simulink model "top_level_algo"  (R2022b)
settings: Solver=FixedStepAuto  StartTime=0.0  StopTime=inf  FixedStep=1e-3  RelTol=1e-3
values from neighbouring files (symbols this model uses):
  clk_period = 8    [Cals.m]
  gear_ratio = 10    [Cals.m]
  update_rate = 0.5    [Cals.m]
  Vdd = 3    [Cals.m]
undefined symbols (not defined in the file or in its folder): sigbuilder_block
libraries: simulink x24, stm32f4xxblockslib x12, embmathops x9, arduinolib x8, dspstat3 x4, dspswit3 x2
(part 3 of 3)

== system top_level_algo/7seg Driver2/HR Encoding/7seg encoder2/If Action Subsystem10 ==
  Action Port : ActionPort  ActionPortLabel=case [ 9 ]:
  Constant : Constant  Value=0x6F
  Out1 : Outport
  wires:
  Constant/1 -> Out1/1

== system top_level_algo/7seg Driver2/HR Encoding/7seg encoder2/If Action Subsystem2 ==
  Action Port : ActionPort  ActionPortLabel=case [ 2 ]:
  Constant : Constant  Value=0x5B
  Out1 : Outport
  wires:
  Constant/1 -> Out1/1

== system top_level_algo/7seg Driver2/HR Encoding/7seg encoder2/If Action Subsystem3 ==
  Action Port : ActionPort  ActionPortLabel=case [ 3 ]:
  Constant : Constant  Value=0x4F
  Out1 : Outport
  wires:
  Constant/1 -> Out1/1

== system top_level_algo/7seg Driver2/HR Encoding/7seg encoder2/If Action Subsystem4 ==
  Action Port : ActionPort  ActionPortLabel=case [ 4 ]:
  Constant : Constant  Value=0x66
  Out1 : Outport
  wires:
  Constant/1 -> Out1/1

== system top_level_algo/7seg Driver2/HR Encoding/7seg encoder2/If Action Subsystem5 ==
  Action Port : ActionPort  ActionPortLabel=case [ 5 ]:
  Constant : Constant  Value=0x6D
  Out1 : Outport
  wires:
  Constant/1 -> Out1/1

== system top_level_algo/7seg Driver2/HR Encoding/7seg encoder2/If Action Subsystem6 ==
  Action Port : ActionPort  ActionPortLabel=case [ 6 ]:
  Constant : Constant  Value=0x7D
  Out1 : Outport
  wires:
  Constant/1 -> Out1/1

== system top_level_algo/7seg Driver2/HR Encoding/7seg encoder2/If Action Subsystem7 ==
  Action Port : ActionPort  ActionPortLabel=case [ 7 ]:
  Constant : Constant  Value=0x07
  Out1 : Outport
  wires:
  Constant/1 -> Out1/1

== system top_level_algo/7seg Driver2/HR Encoding/7seg encoder2/If Action Subsystem8 ==
  Action Port : ActionPort  ActionPortLabel=case [ 8 ]:
  Constant : Constant  Value=0x7F
  Out1 : Outport
  wires:
  Constant/1 -> Out1/1

== system top_level_algo/7seg Driver2/HR Encoding/old encoder3/If Action Subsystem ==
  Action Port : ActionPort
  Constant : Constant  Value=0x3F
  Out1 : Outport
  wires:
  Constant/1 -> Out1/1

== system top_level_algo/7seg Driver2/HR Encoding/old encoder3/If Action Subsystem1 ==
  Action Port : ActionPort
  Constant : Constant  Value=0x06
  Out1 : Outport
  wires:
  Constant/1 -> Out1/1

== system top_level_algo/7seg Driver2/HR Encoding/old encoder3/If Action Subsystem10 ==
  Action Port : ActionPort
  Constant : Constant  Value=0x6F
  Out1 : Outport
  wires:
  Constant/1 -> Out1/1

== system top_level_algo/7seg Driver2/HR Encoding/old encoder3/If Action Subsystem2 ==
  Action Port : ActionPort
  Constant : Constant  Value=0x5B
  Out1 : Outport
  wires:
  Constant/1 -> Out1/1

== system top_level_algo/7seg Driver2/HR Encoding/old encoder3/If Action Subsystem3 ==
  Action Port : ActionPort
  Constant : Constant  Value=0x4F
  Out1 : Outport
  wires:
  Constant/1 -> Out1/1

== system top_level_algo/7seg Driver2/HR Encoding/old encoder3/If Action Subsystem4 ==
  Action Port : ActionPort
  Constant : Constant  Value=0x66
  Out1 : Outport
  wires:
  Constant/1 -> Out1/1

== system top_level_algo/7seg Driver2/HR Encoding/old encoder3/If Action Subsystem5 ==
  Action Port : ActionPort
  Constant : Constant  Value=0x6D
  Out1 : Outport
  wires:
  Constant/1 -> Out1/1

== system top_level_algo/7seg Driver2/HR Encoding/old encoder3/If Action Subsystem6 ==
  Action Port : ActionPort
  Constant : Constant  Value=0x7D
  Out1 : Outport
  wires:
  Constant/1 -> Out1/1

== system top_level_algo/7seg Driver2/HR Encoding/old encoder3/If Action Subsystem7 ==
  Action Port : ActionPort
  Constant : Constant  Value=0x07
  Out1 : Outport
  wires:
  Constant/1 -> Out1/1

== system top_level_algo/7seg Driver2/HR Encoding/old encoder3/If Action Subsystem8 ==
  Action Port : ActionPort
  Constant : Constant  Value=0x7F
  Out1 : Outport
  wires:
  Constant/1 -> Out1/1

== system top_level_algo/Speed up 7seg Driver/HR Encoding/7seg encoder/If Action Subsystem ==
  Action Port : ActionPort  ActionPortLabel=case [ 0 ]:
  Constant : Constant  Value=0x3F
  Out1 : Outport
  wires:
  Constant/1 -> Out1/1

== system top_level_algo/Speed up 7seg Driver/HR Encoding/7seg encoder/If Action Subsystem1 ==
  Action Port : ActionPort  ActionPortLabel=case [ 1 ]:
  Constant : Constant  Value=0x06
  Out1 : Outport
  wires:
  Constant/1 -> Out1/1

== system top_level_algo/Speed up 7seg Driver/HR Encoding/7seg encoder/If Action Subsystem10 ==
  Action Port : ActionPort  ActionPortLabel=case [ 9 ]:
  Constant : Constant  Value=0x6F
  Out1 : Outport
  wires:
  Constant/1 -> Out1/1

== system top_level_algo/Speed up 7seg Driver/HR Encoding/7seg encoder/If Action Subsystem2 ==
  Action Port : ActionPort  ActionPortLabel=case [ 2 ]:
  Constant : Constant  Value=0x5B
  Out1 : Outport
  wires:
  Constant/1 -> Out1/1

== system top_level_algo/Speed up 7seg Driver/HR Encoding/7seg encoder/If Action Subsystem3 ==
  Action Port : ActionPort  ActionPortLabel=case [ 3 ]:
  Constant : Constant  Value=0x4F
  Out1 : Outport
  wires:
  Constant/1 -> Out1/1

== system top_level_algo/Speed up 7seg Driver/HR Encoding/7seg encoder/If Action Subsystem4 ==
  Action Port : ActionPort  ActionPortLabel=case [ 4 ]:
  Constant : Constant  Value=0x66
  Out1 : Outport
  wires:
  Constant/1 -> Out1/1

== system top_level_algo/Speed up 7seg Driver/HR Encoding/7seg encoder/If Action Subsystem5 ==
  Action Port : ActionPort  ActionPortLabel=case [ 5 ]:
  Constant : Constant  Value=0x6D
  Out1 : Outport
  wires:
  Constant/1 -> Out1/1

== system top_level_algo/Speed up 7seg Driver/HR Encoding/7seg encoder/If Action Subsystem6 ==
  Action Port : ActionPort  ActionPortLabel=case [ 6 ]:
  Constant : Constant  Value=0x7D
  Out1 : Outport
  wires:
  Constant/1 -> Out1/1

== system top_level_algo/Speed up 7seg Driver/HR Encoding/7seg encoder/If Action Subsystem7 ==
  Action Port : ActionPort  ActionPortLabel=case [ 7 ]:
  Constant : Constant  Value=0x07
  Out1 : Outport
  wires:
  Constant/1 -> Out1/1

== system top_level_algo/Speed up 7seg Driver/HR Encoding/7seg encoder/If Action Subsystem8 ==
  Action Port : ActionPort  ActionPortLabel=case [ 8 ]:
  Constant : Constant  Value=0x7F
  Out1 : Outport
  wires:
  Constant/1 -> Out1/1

== system top_level_algo/Speed up 7seg Driver/HR Encoding/7seg encoder1/If Action Subsystem ==
  Action Port : ActionPort  ActionPortLabel=case [ 0 ]:
  Constant : Constant  Value=0x3F
  Out1 : Outport
  wires:
  Constant/1 -> Out1/1

== system top_level_algo/Speed up 7seg Driver/HR Encoding/7seg encoder1/If Action Subsystem1 ==
  Action Port : ActionPort  ActionPortLabel=case [ 1 ]:
  Constant : Constant  Value=0x06
  Out1 : Outport
  wires:
  Constant/1 -> Out1/1

== system top_level_algo/Speed up 7seg Driver/HR Encoding/7seg encoder1/If Action Subsystem10 ==
  Action Port : ActionPort  ActionPortLabel=case [ 9 ]:
  Constant : Constant  Value=0x6F
  Out1 : Outport
  wires:
  Constant/1 -> Out1/1

== system top_level_algo/Speed up 7seg Driver/HR Encoding/7seg encoder1/If Action Subsystem2 ==
  Action Port : ActionPort  ActionPortLabel=case [ 2 ]:
  Constant : Constant  Value=0x5B
  Out1 : Outport
  wires:
  Constant/1 -> Out1/1

== system top_level_algo/Speed up 7seg Driver/HR Encoding/7seg encoder1/If Action Subsystem3 ==
  Action Port : ActionPort  ActionPortLabel=case [ 3 ]:
  Constant : Constant  Value=0x4F
  Out1 : Outport
  wires:
  Constant/1 -> Out1/1

== system top_level_algo/Speed up 7seg Driver/HR Encoding/7seg encoder1/If Action Subsystem4 ==
  Action Port : ActionPort  ActionPortLabel=case [ 4 ]:
  Constant : Constant  Value=0x66
  Out1 : Outport
  wires:
  Constant/1 -> Out1/1

== system top_level_algo/Speed up 7seg Driver/HR Encoding/7seg encoder1/If Action Subsystem5 ==
  Action Port : ActionPort  ActionPortLabel=case [ 5 ]:
  Constant : Constant  Value=0x6D
  Out1 : Outport
  wires:
  Constant/1 -> Out1/1

== system top_level_algo/Speed up 7seg Driver/HR Encoding/7seg encoder1/If Action Subsystem6 ==
  Action Port : ActionPort  ActionPortLabel=case [ 6 ]:
  Constant : Constant  Value=0x7D
  Out1 : Outport
  wires:
  Constant/1 -> Out1/1

== system top_level_algo/Speed up 7seg Driver/HR Encoding/7seg encoder1/If Action Subsystem7 ==
  Action Port : ActionPort  ActionPortLabel=case [ 7 ]:
  Constant : Constant  Value=0x07
  Out1 : Outport
  wires:
  Constant/1 -> Out1/1

== system top_level_algo/Speed up 7seg Driver/HR Encoding/7seg encoder1/If Action Subsystem8 ==
  Action Port : ActionPort  ActionPortLabel=case [ 8 ]:
  Constant : Constant  Value=0x7F
  Out1 : Outport
  wires:
  Constant/1 -> Out1/1

== system top_level_algo/Speed up 7seg Driver/HR Encoding/7seg encoder2/If Action Subsystem ==
  Action Port : ActionPort  ActionPortLabel=case [ 0 ]:
  Constant : Constant  Value=0x3F
  Out1 : Outport
  wires:
  Constant/1 -> Out1/1

== system top_level_algo/Speed up 7seg Driver/HR Encoding/7seg encoder2/If Action Subsystem1 ==
  Action Port : ActionPort  ActionPortLabel=case [ 1 ]:
  Constant : Constant  Value=0x06
  Out1 : Outport
  wires:
  Constant/1 -> Out1/1

== system top_level_algo/Speed up 7seg Driver/HR Encoding/7seg encoder2/If Action Subsystem10 ==
  Action Port : ActionPort  ActionPortLabel=case [ 9 ]:
  Constant : Constant  Value=0x6F
  Out1 : Outport
  wires:
  Constant/1 -> Out1/1

== system top_level_algo/Speed up 7seg Driver/HR Encoding/7seg encoder2/If Action Subsystem2 ==
  Action Port : ActionPort  ActionPortLabel=case [ 2 ]:
  Constant : Constant  Value=0x5B
  Out1 : Outport
  wires:
  Constant/1 -> Out1/1

== system top_level_algo/Speed up 7seg Driver/HR Encoding/7seg encoder2/If Action Subsystem3 ==
  Action Port : ActionPort  ActionPortLabel=case [ 3 ]:
  Constant : Constant  Value=0x4F
  Out1 : Outport
  wires:
  Constant/1 -> Out1/1

== system top_level_algo/Speed up 7seg Driver/HR Encoding/7seg encoder2/If Action Subsystem4 ==
  Action Port : ActionPort  ActionPortLabel=case [ 4 ]:
  Constant : Constant  Value=0x66
  Out1 : Outport
  wires:
  Constant/1 -> Out1/1

== system top_level_algo/Speed up 7seg Driver/HR Encoding/7seg encoder2/If Action Subsystem5 ==
  Action Port : ActionPort  ActionPortLabel=case [ 5 ]:
  Constant : Constant  Value=0x6D
  Out1 : Outport
  wires:
  Constant/1 -> Out1/1

== system top_level_algo/Speed up 7seg Driver/HR Encoding/7seg encoder2/If Action Subsystem6 ==
  Action Port : ActionPort  ActionPortLabel=case [ 6 ]:
  Constant : Constant  Value=0x7D
  Out1 : Outport
  wires:
  Constant/1 -> Out1/1

== system top_level_algo/Speed up 7seg Driver/HR Encoding/7seg encoder2/If Action Subsystem7 ==
  Action Port : ActionPort  ActionPortLabel=case [ 7 ]:
  Constant : Constant  Value=0x07
  Out1 : Outport
  wires:
  Constant/1 -> Out1/1

== system top_level_algo/Speed up 7seg Driver/HR Encoding/7seg encoder2/If Action Subsystem8 ==
  Action Port : ActionPort  ActionPortLabel=case [ 8 ]:
  Constant : Constant  Value=0x7F
  Out1 : Outport
  wires:
  Constant/1 -> Out1/1

== system top_level_algo/Speed up 7seg Driver/HR Encoding/old encoder3/If Action Subsystem ==
  Action Port : ActionPort
  Constant : Constant  Value=0x3F
  Out1 : Outport
  wires:
  Constant/1 -> Out1/1

== system top_level_algo/Speed up 7seg Driver/HR Encoding/old encoder3/If Action Subsystem1 ==
  Action Port : ActionPort
  Constant : Constant  Value=0x06
  Out1 : Outport
  wires:
  Constant/1 -> Out1/1

== system top_level_algo/Speed up 7seg Driver/HR Encoding/old encoder3/If Action Subsystem10 ==
  Action Port : ActionPort
  Constant : Constant  Value=0x6F
  Out1 : Outport
  wires:
  Constant/1 -> Out1/1

== system top_level_algo/Speed up 7seg Driver/HR Encoding/old encoder3/If Action Subsystem2 ==
  Action Port : ActionPort
  Constant : Constant  Value=0x5B
  Out1 : Outport
  wires:
  Constant/1 -> Out1/1

== system top_level_algo/Speed up 7seg Driver/HR Encoding/old encoder3/If Action Subsystem3 ==
  Action Port : ActionPort
  Constant : Constant  Value=0x4F
  Out1 : Outport
  wires:
  Constant/1 -> Out1/1

== system top_level_algo/Speed up 7seg Driver/HR Encoding/old encoder3/If Action Subsystem4 ==
  Action Port : ActionPort
  Constant : Constant  Value=0x66
  Out1 : Outport
  wires:
  Constant/1 -> Out1/1

== system top_level_algo/Speed up 7seg Driver/HR Encoding/old encoder3/If Action Subsystem5 ==
  Action Port : ActionPort
  Constant : Constant  Value=0x6D
  Out1 : Outport
  wires:
  Constant/1 -> Out1/1

== system top_level_algo/Speed up 7seg Driver/HR Encoding/old encoder3/If Action Subsystem6 ==
  Action Port : ActionPort
  Constant : Constant  Value=0x7D
  Out1 : Outport
  wires:
  Constant/1 -> Out1/1

== system top_level_algo/Speed up 7seg Driver/HR Encoding/old encoder3/If Action Subsystem7 ==
  Action Port : ActionPort
  Constant : Constant  Value=0x07
  Out1 : Outport
  wires:
  Constant/1 -> Out1/1

== system top_level_algo/Speed up 7seg Driver/HR Encoding/old encoder3/If Action Subsystem8 ==
  Action Port : ActionPort
  Constant : Constant  Value=0x7F
  Out1 : Outport
  wires:
  Constant/1 -> Out1/1

== system top_level_algo/Speed up 7seg Driver1/HR Encoding/7seg encoder/If Action Subsystem ==
  Action Port : ActionPort  ActionPortLabel=case [ 0 ]:
  Constant : Constant  Value=0x3F
  Out1 : Outport
  wires:
  Constant/1 -> Out1/1

== system top_level_algo/Speed up 7seg Driver1/HR Encoding/7seg encoder/If Action Subsystem1 ==
  Action Port : ActionPort  ActionPortLabel=case [ 1 ]:
  Constant : Constant  Value=0x06
  Out1 : Outport
  wires:
  Constant/1 -> Out1/1

== system top_level_algo/Speed up 7seg Driver1/HR Encoding/7seg encoder/If Action Subsystem10 ==
  Action Port : ActionPort  ActionPortLabel=case [ 9 ]:
  Constant : Constant  Value=0x6F
  Out1 : Outport
  wires:
  Constant/1 -> Out1/1

== system top_level_algo/Speed up 7seg Driver1/HR Encoding/7seg encoder/If Action Subsystem2 ==
  Action Port : ActionPort  ActionPortLabel=case [ 2 ]:
  Constant : Constant  Value=0x5B
  Out1 : Outport
  wires:
  Constant/1 -> Out1/1

== system top_level_algo/Speed up 7seg Driver1/HR Encoding/7seg encoder/If Action Subsystem3 ==
  Action Port : ActionPort  ActionPortLabel=case [ 3 ]:
  Constant : Constant  Value=0x4F
  Out1 : Outport
  wires:
  Constant/1 -> Out1/1

== system top_level_algo/Speed up 7seg Driver1/HR Encoding/7seg encoder/If Action Subsystem4 ==
  Action Port : ActionPort  ActionPortLabel=case [ 4 ]:
  Constant : Constant  Value=0x66
  Out1 : Outport
  wires:
  Constant/1 -> Out1/1

== system top_level_algo/Speed up 7seg Driver1/HR Encoding/7seg encoder/If Action Subsystem5 ==
  Action Port : ActionPort  ActionPortLabel=case [ 5 ]:
  Constant : Constant  Value=0x6D
  Out1 : Outport
  wires:
  Constant/1 -> Out1/1

== system top_level_algo/Speed up 7seg Driver1/HR Encoding/7seg encoder/If Action Subsystem6 ==
  Action Port : ActionPort  ActionPortLabel=case [ 6 ]:
  Constant : Constant  Value=0x7D
  Out1 : Outport
  wires:
  Constant/1 -> Out1/1

== system top_level_algo/Speed up 7seg Driver1/HR Encoding/7seg encoder/If Action Subsystem7 ==
  Action Port : ActionPort  ActionPortLabel=case [ 7 ]:
  Constant : Constant  Value=0x07
  Out1 : Outport
  wires:
  Constant/1 -> Out1/1

== system top_level_algo/Speed up 7seg Driver1/HR Encoding/7seg encoder/If Action Subsystem8 ==
  Action Port : ActionPort  ActionPortLabel=case [ 8 ]:
  Constant : Constant  Value=0x7F
  Out1 : Outport
  wires:
  Constant/1 -> Out1/1

== system top_level_algo/Speed up 7seg Driver1/HR Encoding/7seg encoder1/If Action Subsystem ==
  Action Port : ActionPort  ActionPortLabel=case [ 0 ]:
  Constant : Constant  Value=0x3F
  Out1 : Outport
  wires:
  Constant/1 -> Out1/1

== system top_level_algo/Speed up 7seg Driver1/HR Encoding/7seg encoder1/If Action Subsystem1 ==
  Action Port : ActionPort  ActionPortLabel=case [ 1 ]:
  Constant : Constant  Value=0x06
  Out1 : Outport
  wires:
  Constant/1 -> Out1/1

== system top_level_algo/Speed up 7seg Driver1/HR Encoding/7seg encoder1/If Action Subsystem10 ==
  Action Port : ActionPort  ActionPortLabel=case [ 9 ]:
  Constant : Constant  Value=0x6F
  Out1 : Outport
  wires:
  Constant/1 -> Out1/1

== system top_level_algo/Speed up 7seg Driver1/HR Encoding/7seg encoder1/If Action Subsystem2 ==
  Action Port : ActionPort  ActionPortLabel=case [ 2 ]:
  Constant : Constant  Value=0x5B
  Out1 : Outport
  wires:
  Constant/1 -> Out1/1

== system top_level_algo/Speed up 7seg Driver1/HR Encoding/7seg encoder1/If Action Subsystem3 ==
  Action Port : ActionPort  ActionPortLabel=case [ 3 ]:
  Constant : Constant  Value=0x4F
  Out1 : Outport
  wires:
  Constant/1 -> Out1/1

== system top_level_algo/Speed up 7seg Driver1/HR Encoding/7seg encoder1/If Action Subsystem4 ==
  Action Port : ActionPort  ActionPortLabel=case [ 4 ]:
  Constant : Constant  Value=0x66
  Out1 : Outport
  wires:
  Constant/1 -> Out1/1

== system top_level_algo/Speed up 7seg Driver1/HR Encoding/7seg encoder1/If Action Subsystem5 ==
  Action Port : ActionPort  ActionPortLabel=case [ 5 ]:
  Constant : Constant  Value=0x6D
  Out1 : Outport
  wires:
  Constant/1 -> Out1/1

== system top_level_algo/Speed up 7seg Driver1/HR Encoding/7seg encoder1/If Action Subsystem6 ==
  Action Port : ActionPort  ActionPortLabel=case [ 6 ]:
  Constant : Constant  Value=0x7D
  Out1 : Outport
  wires:
  Constant/1 -> Out1/1

== system top_level_algo/Speed up 7seg Driver1/HR Encoding/7seg encoder1/If Action Subsystem7 ==
  Action Port : ActionPort  ActionPortLabel=case [ 7 ]:
  Constant : Constant  Value=0x07
  Out1 : Outport
  wires:
  Constant/1 -> Out1/1

== system top_level_algo/Speed up 7seg Driver1/HR Encoding/7seg encoder1/If Action Subsystem8 ==
  Action Port : ActionPort  ActionPortLabel=case [ 8 ]:
  Constant : Constant  Value=0x7F
  Out1 : Outport
  wires:
  Constant/1 -> Out1/1

== system top_level_algo/Speed up 7seg Driver1/HR Encoding/7seg encoder2/If Action Subsystem ==
  Action Port : ActionPort  ActionPortLabel=case [ 0 ]:
  Constant : Constant  Value=0x3F
  Out1 : Outport
  wires:
  Constant/1 -> Out1/1

== system top_level_algo/Speed up 7seg Driver1/HR Encoding/7seg encoder2/If Action Subsystem1 ==
  Action Port : ActionPort  ActionPortLabel=case [ 1 ]:
  Constant : Constant  Value=0x06
  Out1 : Outport
  wires:
  Constant/1 -> Out1/1

== system top_level_algo/Speed up 7seg Driver1/HR Encoding/7seg encoder2/If Action Subsystem10 ==
  Action Port : ActionPort  ActionPortLabel=case [ 9 ]:
  Constant : Constant  Value=0x6F
  Out1 : Outport
  wires:
  Constant/1 -> Out1/1

== system top_level_algo/Speed up 7seg Driver1/HR Encoding/7seg encoder2/If Action Subsystem2 ==
  Action Port : ActionPort  ActionPortLabel=case [ 2 ]:
  Constant : Constant  Value=0x5B
  Out1 : Outport
  wires:
  Constant/1 -> Out1/1

== system top_level_algo/Speed up 7seg Driver1/HR Encoding/7seg encoder2/If Action Subsystem3 ==
  Action Port : ActionPort  ActionPortLabel=case [ 3 ]:
  Constant : Constant  Value=0x4F
  Out1 : Outport
  wires:
  Constant/1 -> Out1/1

== system top_level_algo/Speed up 7seg Driver1/HR Encoding/7seg encoder2/If Action Subsystem4 ==
  Action Port : ActionPort  ActionPortLabel=case [ 4 ]:
  Constant : Constant  Value=0x66
  Out1 : Outport
  wires:
  Constant/1 -> Out1/1

== system top_level_algo/Speed up 7seg Driver1/HR Encoding/7seg encoder2/If Action Subsystem5 ==
  Action Port : ActionPort  ActionPortLabel=case [ 5 ]:
  Constant : Constant  Value=0x6D
  Out1 : Outport
  wires:
  Constant/1 -> Out1/1

== system top_level_algo/Speed up 7seg Driver1/HR Encoding/7seg encoder2/If Action Subsystem6 ==
  Action Port : ActionPort  ActionPortLabel=case [ 6 ]:
  Constant : Constant  Value=0x7D
  Out1 : Outport
  wires:
  Constant/1 -> Out1/1

== system top_level_algo/Speed up 7seg Driver1/HR Encoding/7seg encoder2/If Action Subsystem7 ==
  Action Port : ActionPort  ActionPortLabel=case [ 7 ]:
  Constant : Constant  Value=0x07
  Out1 : Outport
  wires:
  Constant/1 -> Out1/1

== system top_level_algo/Speed up 7seg Driver1/HR Encoding/7seg encoder2/If Action Subsystem8 ==
  Action Port : ActionPort  ActionPortLabel=case [ 8 ]:
  Constant : Constant  Value=0x7F
  Out1 : Outport
  wires:
  Constant/1 -> Out1/1

== system top_level_algo/Speed up 7seg Driver1/HR Encoding/old encoder3/If Action Subsystem ==
  Action Port : ActionPort
  Constant : Constant  Value=0x3F
  Out1 : Outport
  wires:
  Constant/1 -> Out1/1

== system top_level_algo/Speed up 7seg Driver1/HR Encoding/old encoder3/If Action Subsystem1 ==
  Action Port : ActionPort
  Constant : Constant  Value=0x06
  Out1 : Outport
  wires:
  Constant/1 -> Out1/1

== system top_level_algo/Speed up 7seg Driver1/HR Encoding/old encoder3/If Action Subsystem10 ==
  Action Port : ActionPort
  Constant : Constant  Value=0x6F
  Out1 : Outport
  wires:
  Constant/1 -> Out1/1

== system top_level_algo/Speed up 7seg Driver1/HR Encoding/old encoder3/If Action Subsystem2 ==
  Action Port : ActionPort
  Constant : Constant  Value=0x5B
  Out1 : Outport
  wires:
  Constant/1 -> Out1/1

== system top_level_algo/Speed up 7seg Driver1/HR Encoding/old encoder3/If Action Subsystem3 ==
  Action Port : ActionPort
  Constant : Constant  Value=0x4F
  Out1 : Outport
  wires:
  Constant/1 -> Out1/1

== system top_level_algo/Speed up 7seg Driver1/HR Encoding/old encoder3/If Action Subsystem4 ==
  Action Port : ActionPort
  Constant : Constant  Value=0x66
  Out1 : Outport
  wires:
  Constant/1 -> Out1/1

== system top_level_algo/Speed up 7seg Driver1/HR Encoding/old encoder3/If Action Subsystem5 ==
  Action Port : ActionPort
  Constant : Constant  Value=0x6D
  Out1 : Outport
  wires:
  Constant/1 -> Out1/1

== system top_level_algo/Speed up 7seg Driver1/HR Encoding/old encoder3/If Action Subsystem6 ==
  Action Port : ActionPort
  Constant : Constant  Value=0x7D
  Out1 : Outport
  wires:
  Constant/1 -> Out1/1

== system top_level_algo/Speed up 7seg Driver1/HR Encoding/old encoder3/If Action Subsystem7 ==
  Action Port : ActionPort
  Constant : Constant  Value=0x07
  Out1 : Outport
  wires:
  Constant/1 -> Out1/1

== system top_level_algo/Speed up 7seg Driver1/HR Encoding/old encoder3/If Action Subsystem8 ==
  Action Port : ActionPort
  Constant : Constant  Value=0x7F
  Out1 : Outport
  wires:
  Constant/1 -> Out1/1

== stateflow chart top_level_algo/7seg Driver/Subsystem/ClockLogic ==
  state START
    counter = 0;
    CLK = 0;
  state HIGH
    entry:
    CLK = 1;
  state LOW
    entry:
    CLK = 0;
    counter = counter +1;
  state WAIT
  (default) -> START
  START -> WAIT : [Set == 1]
  LOW -> START [order 1] : [counter == 36]
  LOW -> HIGH [order 2] : after(10,msec)
  WAIT -> HIGH : after(10,msec)
  HIGH -> LOW : after(10,msec)
  data: CLK output; Set input; counter local

== stateflow chart top_level_algo/7seg Driver/Subsystem/DataLogic ==
  state LOAD
    entry:
    data = 0;
    Holder = HR;
  state WAITING
  state Wait
  state MASK
    entry:
    data = bitand(Holder, 1);
  state START
    entry:
    data = 1;
  state CHECK
    entry:
    Holder = bitshift(Holder,-1);
  (default) -> LOAD
  WAITING -> LOAD : after(10,msec)
  LOAD -> Wait : [Set == 1]
  CHECK -> WAITING [order 1] : [Holder == 0]
  Wait -> START : after(5,msec)
  START -> MASK : after(20,msec)
  CHECK -> MASK [order 2] : after(10,msec)
  MASK -> CHECK : after(10,msec)
  data: HR input; data output uint32; Set input; Holder local

== stateflow chart top_level_algo/Chart ==
  state Start
    entry:
    my_count = 111;
  state Counting
    entry:
    my_count = my_count + 1;
  (default) -> Start
  Start -> Counting
  Counting -> Counting : after(300,msec)
  data: my_count output

== stateflow chart top_level_algo/Speed up 7seg Driver/ClockLogic ==
  state START
    counter = 0;
    CLK = 0;
  state WAIT
  state HIGH
    entry:
    CLK = 1;
  state LOW
    entry:
    CLK = 0;
    counter = counter +1;
  (default) -> START
  START -> WAIT : [Set == 1]
  LOW -> START [order 1] : [counter == 36]
  LOW -> HIGH [order 2] : after(clk_period/2,msec)
  WAIT -> HIGH : after(clk_period/2,msec)
  HIGH -> LOW : after(clk_period/2,msec)
  data: CLK output; Set input; counter local; clk_period parameter double

== stateflow chart top_level_algo/Speed up 7seg Driver/DataLogic ==
  state LOAD
    entry:
    data = 0;
    Holder = HR;
  state HOLD
    entry:
    data = 0;
  state WAITING
  state Wait
  state MASK
    entry:
    data = bitand(Holder, 1);
  state START
    entry:
    data = 1;
  state CHECK
    entry:
    Holder = bitshift(Holder,-1);
  (default) -> LOAD
  HOLD -> LOAD : [Set == 0]
  WAITING -> HOLD : after(clk_period/2,msec)
  LOAD -> Wait : [Set == 1]
  CHECK -> WAITING [order 1] : [Holder == 0]
  Wait -> START : after(clk_period/4,msec)
  START -> MASK : after(clk_period,msec)
  CHECK -> MASK [order 2] : after(clk_period/2,msec)
  MASK -> CHECK : after(clk_period/2,msec)
  data: HR input; data output uint32; Set input; Holder local; clk_period parameter

== stateflow chart top_level_algo/7seg Driver2/Subsystem/ClockLogic ==
  state START
    counter = 0;
    CLK = 0;
  state HIGH
    entry:
    CLK = 1;
  state LOW
    entry:
    CLK = 0;
    counter = counter +1;
  state WAIT
  (default) -> START
  START -> WAIT : [Set == 1]
  LOW -> START [order 1] : [counter == 36]
  LOW -> HIGH [order 2] : after(10,msec)
  WAIT -> HIGH : after(10,msec)
  HIGH -> LOW : after(10,msec)
  data: CLK output; Set input; counter local

== stateflow chart top_level_algo/7seg Driver2/Subsystem/DataLogic ==
  state LOAD
    entry:
    data = 0;
    Holder = HR;
  state WAITING
  state Wait
  state MASK
    entry:
    data = bitand(Holder, 1);
  state START
    entry:
    data = 1;
  state CHECK
    entry:
    Holder = bitshift(Holder,-1);
  (default) -> LOAD
  WAITING -> LOAD : after(10,msec)
  LOAD -> Wait : [Set == 1]
  CHECK -> WAITING [order 1] : [Holder == 0]
  Wait -> START : after(5,msec)
  START -> MASK : after(20,msec)
  CHECK -> MASK [order 2] : after(10,msec)
  MASK -> CHECK : after(10,msec)
  data: HR input; data output uint32; Set input; Holder local

== stateflow chart top_level_algo/Compression Detection/Chart1 ==
  state INIT
    entry:
    sumDetect = 0;
    lastTs = 0;
    paceDetect = 0;
  state First
    entry:
    sumDetect = 0;
    lastTs = newTs;
  state Counting
    entry:
    outNew = newTs - lastTs;
    paceDetect = (60/(newTs-lastTs)); %1/period * 60 (to BPM)
    lastTs = newTs;
    outTs = lastTs;
  (default) -> INIT
  Counting -> INIT [order 2] : after(2,sec)
  INIT -> First : [detect == true]{newTs = clTime;}
  First -> Counting : [after(50,msec)&&[detect == true]]{newTs = clTime;}
  Counting -> Counting [order 1] : [(after(10,msec)&&[detect == true])]{newTs = clTime;}
  data: clTime input; detect input boolean; paceDetect output double; sumDetect local; newTs local double; lastTs local double; outTs output; outNew output

== stateflow chart top_level_algo/Chart1 ==
  state Start
    entry:
    my_count = 0;
  state Counting
    entry:
    my_count = my_count + 1;
  (default) -> Start
  Counting -> Start [order 2] : [my_count == 201]
  Start -> Counting
  Counting -> Counting [order 1] : after(1000,msec)
  data: my_count output

== stateflow chart top_level_algo/Speed up 7seg Driver1/ClockLogic ==
  state START
    counter = 0;
    CLK = 0;
  state WAIT
  state HIGH
    entry:
    CLK = 1;
  state LOW
    entry:
    CLK = 0;
    counter = counter +1;
  (default) -> START
  START -> WAIT : [Set == 1]
  LOW -> START [order 1] : [counter == 36]
  LOW -> HIGH [order 2] : after(clk_period/2,msec)
  WAIT -> HIGH : after(clk_period/2,msec)
  HIGH -> LOW : after(clk_period/2,msec)
  data: CLK output; Set input; counter local; clk_period parameter double

== stateflow chart top_level_algo/Speed up 7seg Driver1/DataLogic ==
  state LOAD
    entry:
    data = 0;
    Holder = HR;
  state HOLD
    entry:
    data = 0;
  state WAITING
  state Wait
  state MASK
    entry:
    data = bitand(Holder, 1);
  state START
    entry:
    data = 1;
  state CHECK
    entry:
    Holder = bitshift(Holder,-1);
  (default) -> LOAD
  HOLD -> LOAD : [Set == 0]
  WAITING -> HOLD : after(clk_period/2,msec)
  LOAD -> Wait : [Set == 1]
  CHECK -> WAITING [order 1] : [Holder == 0]
  Wait -> START : after(clk_period/4,msec)
  START -> MASK : after(clk_period,msec)
  CHECK -> MASK [order 2] : after(clk_period/2,msec)
  MASK -> CHECK : after(clk_period/2,msec)
  data: HR input; data output uint32; Set input; Holder local; clk_period parameter

== stateflow chart top_level_algo/MinMax/sample and hold ==
  state Init
    entry:
    displacement = 0;
  state Holding
    entry:
    displacement = max;
  (default) -> Init
  Init -> Holding : [read == true]
  Holding -> Holding : [read == true]
  data: max input; read input; displacement output

== stateflow chart top_level_algo/MinMax/sample and hold1 ==
  state Init
    entry:
    displacement = 0;
  state Holding
    entry:
    displacement = max;
  (default) -> Init
  Init -> Holding : [read == true]
  Holding -> Holding : [read == true]
  data: max input; read input; displacement output

== stateflow chart top_level_algo/Hardware Hiding/timer ==
  state Starting
    entry:
    measure_period = 0;
  state Finished
    entry:
    baseline = data;
    measure_period = 1;
  (default) -> Starting
  Starting -> Finished : after(2000,msec)
  data: baseline output; measure_period output; data input

== stateflow chart top_level_algo/Compression Detection/Chart ==
  state INIT
    entry:
    count = 0;
    comp = 0;
    rate = 0;
    zero = 0;
    first = 0;
    second = 0;
    third = 0;
    fourth = 0;
  state ONE
    entry:
    first = my_time;
  state DETECTION
    entry:
    comp = comp + 1;
    %%last_count  =count;
    last_count = my_time;
    rate = comp *60/(my_time - zero);
  state POLLING
    entry:
    %%count = my_time;
  state Wait
    entry:
    zero = my_time;
    last_count = my_time;
  state TWO
    entry:
    second = my_time;
  state THREE
    entry:
    third = my_time;
  state FOUR
    entry:
    fourth = my_time;
  state SHORTEN
    entry:
    %%count = count - first;
    rate = comp *60/(my_time - zero);
    last_count  = my_time;
    zero = first;
    first = second;
    second = third;
    third = fourth;
    fourth = my_time;
  (junction 41) -> (junction 24)
  (default) -> INIT
  DETECTION -> INIT [commented out] : [my_time - last_count > 10]
  POLLING -> INIT [order 2] : [my_time - last_count > 4]
  INIT -> Wait : [detect==true]
  POLLING -> POLLING [commented out] : after(200,msec)
  DETECTION -> ONE [order 2] : [first==0]
  ONE -> (junction 41)
  DETECTION -> TWO [order 3] : [first && second==0]
  POLLING -> DETECTION [order 1] : [detect && comp <= 3]
  Wait -> POLLING : [~detect]
  DETECTION -> THREE [order 4] : [first && second && third==0]
  (junction 24) -> POLLING : [~detect]
  TWO -> (junction 41)
  SHORTEN -> POLLING : [~detect]
  POLLING -> SHORTEN [order 3] : [detect && comp >3]
  DETECTION -> FOUR [order 1] : [first && second && third && fourth==0]
  THREE -> (junction 41)
  FOUR -> (junction 41)
  data: my_time input; detect input; rate output; count local; comp local; last_count local; first local; second local; third local; fourth local; zero local
